simulink model "spring_damper_mass"  (R2025a)
settings: Solver=VariableStepAuto  StartTime=0.0  StopTime=10.0  RelTol=1e-3
undefined symbols (not defined in the file): robot, susp, world
settings Model: Creator=yaremadzulynsky  LastModifiedBy=yaremadzulynsky

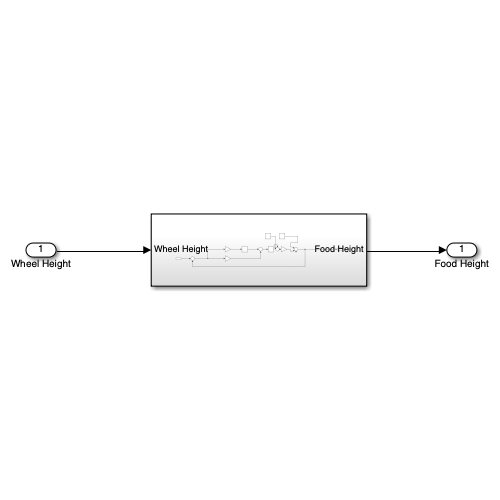
[thumbnail: Simulink's stored preview of the top-level diagram]
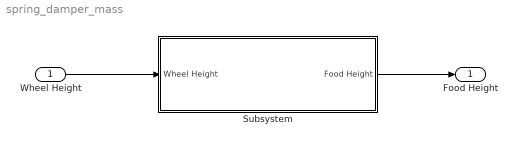
== system spring_damper_mass ==
  Wheel Height : Inport
  Subsystem : Subsystem
  Food Height : Outport
  wires:
  Wheel Height/1 -> Subsystem/1(Wheel Height)
  Subsystem/1(Food Height) -> Food Height/1

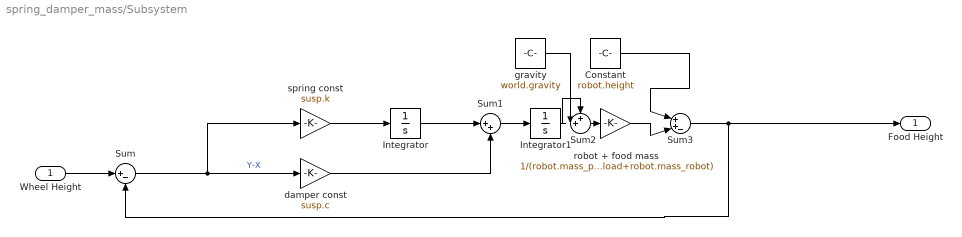
== system spring_damper_mass/Subsystem ==
  Wheel Height : Inport
  Constant : Constant  Value=robot.height
  Integrator : Integrator
  Integrator1 : Integrator
  Sum : Sum  Inputs=|+-
  Sum1 : Sum  Inputs=|++
  Sum2 : Sum  Inputs=++|
  Sum3 : Sum  Inputs=|++-
  damper const : Gain  Gain=susp.c
  gravity : Constant  Value=world.gravity
  robot + food mass : Gain  Gain=1/(robot.mass_payload+robot.mass_robot)
  spring const : Gain  Gain=susp.k
  Food Height : Outport
  wires:
  damper const/1 -> Sum1/2
  spring const/1 -> Integrator/1
  Integrator/1 -> Sum1/1
  Sum/1 -> damper const/1, spring const/1  "Y-X"
  Sum3/1 -> Food Height/1, Sum/2
  Wheel Height/1 -> Sum/1
  Sum1/1 -> Integrator1/1
  gravity/1 -> Sum2/2
  robot + food mass/1 -> Sum3/2
  Constant/1 -> Sum3/1
  Integrator1/1 -> Sum2/1
  Sum2/1 -> robot + food mass/1
